simulink model "soc_dvbs2_hostUDPReceive"  (R2025b)
settings: Solver=VariableStepAuto  StartTime=0.0  StopTime=inf  RelTol=1e-3
values from neighbouring files (symbols this model uses):
  Rsym = 4e6    (= 4000000)    [soc_dvbs2_init.m]
libraries: dspnetwork x2, hdlsllib x2
settings Model: DataTypeOverride=Off  SimulationMode=accelerator  Creator=The MathWorks, Inc.  LastModifiedBy=The MathWorks, Inc.
settings SolverCC: MaxZcPerStep=1.0
settings OptimizationCC: BlockReduction=off  ConditionallyExecuteInputs=off  DefaultParameterBehavior=Inlined  ReuseModelBlockBuffer=off
settings DebuggingCC: AlgebraicLoopMsg=error  SingleTaskRateTransMsg=error  UnconnectedInputMsg=warning  UnconnectedOutputMsg=warning  UnconnectedLineMsg=warning  SubsystemReferenceDiagnosticForUnitTest=warning
settings HardwareCC: ProdBitPerPointer=32.0  ProdBitPerSizeT=32.0  ProdBitPerPtrDiffT=32.0  ProdLargestAtomicFloat=None  ProdIntDivRoundTo=Undefined  ProdEndianess=Unspecified  ProdWordSize=32.0  ProdHWDeviceType=ASIC/FPGA->ASIC/FPGA  TargetBitPerLong=64.0  TargetBitPerPointer=64.0  TargetBitPerSizeT=64.0  TargetBitPerPtrDiffT=64.0  TargetLongLongMode=on  TargetIntDivRoundTo=Zero  TargetEndianess=LittleEndian  TargetWordSize=64.0  TargetHWDeviceType=Custom Processor->MATLAB Host Computer  ProdEqTarget=off
settings ModelReferenceCC: EnableRefExpFcnMdlSchedulingChecks=on
settings RTWCC: GPUComputeCapability=3.5  DLArmComputeVersion=19.05

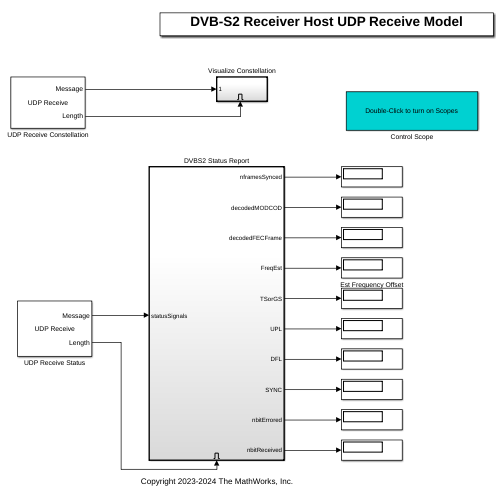
[thumbnail: Simulink's stored preview of the top-level diagram]
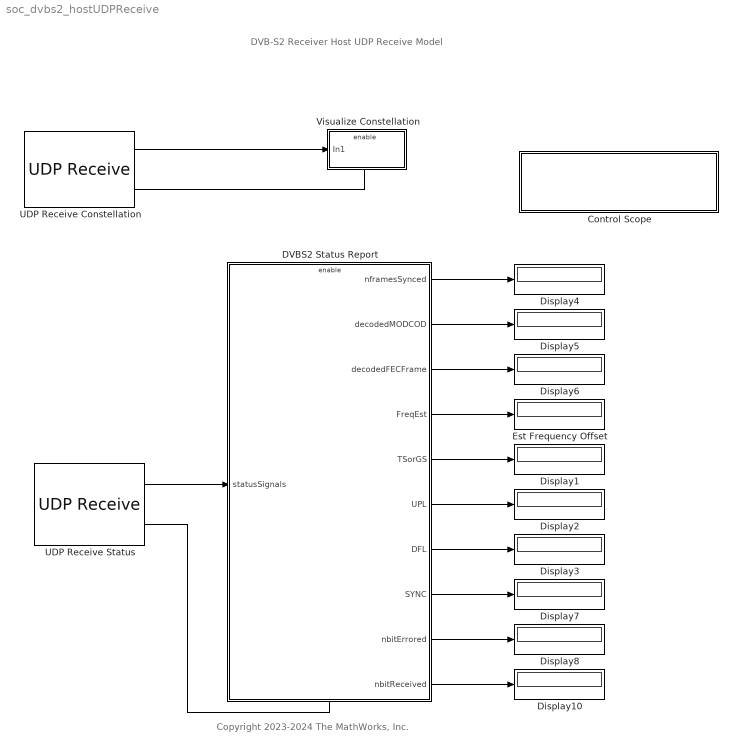
== system soc_dvbs2_hostUDPReceive ==
  note: DVB-S2 Receiver Host UDP Receive Model
  note: Copyright 2023-2024 The MathWorks, Inc.
  Control Scope : Subsystem
      settings: OpenFcn=|
      | ctrl = true;
      | hScopeConfig = get_param([gcs '/Visualize Constellation/Constellation Diagram'],'ScopeConfiguration');
      | hScopeConfig.Visible = ctrl;
      | clear hScopeConfig ctrl;
      mask Display: disp('Double-Click to turn on Scopes');
  DVBS2 Status Report : Subsystem
  Display{1..8,10} (9 alike) : Display
      Display7 settings: Format=hex (Stored Integer)
  Est Frequency Offset : Display
  UDP Receive Constellation : dspnetwork/UDP Receive  localURL='0.0.0.0'  localPort=25000  remoteURL='0.0.0.0'  remotePort=-1  recvBufferSize=8192  dims=2048  signalDatatype=uint32  isComplex=off  isVarSize=off  showBlockingTime=off  blockingTime=0  sampletime=1e-3  blockPlatform=[]
  UDP Receive Status : dspnetwork/UDP Receive  localURL='0.0.0.0'  localPort=25001  remoteURL='0.0.0.0'  remotePort=-1  recvBufferSize=8192  dims=10  signalDatatype=uint32  isComplex=off  isVarSize=off  showBlockingTime=off  blockingTime=0  sampletime=1e-3  blockPlatform=[]
  Visualize Constellation : Subsystem
  wires:
  DVBS2 Status Report/3(decodedFECFrame) -> Display6/1
  DVBS2 Status Report/4(FreqEst) -> Est Frequency Offset/1
  UDP Receive Constellation/1 -> Visualize Constellation/1(In1)
  UDP Receive Status/1 -> DVBS2 Status Report/1(statusSignals)
  DVBS2 Status Report/2(decodedMODCOD) -> Display5/1
  DVBS2 Status Report/1(nframesSynced) -> Display4/1
  UDP Receive Constellation/2 -> Visualize Constellation/Enable
  UDP Receive Status/2 -> DVBS2 Status Report/Enable
  DVBS2 Status Report/5(TSorGS) -> Display1/1
  DVBS2 Status Report/6(UPL) -> Display2/1
  DVBS2 Status Report/7(DFL) -> Display3/1
  DVBS2 Status Report/8(SYNC) -> Display7/1
  DVBS2 Status Report/9(nbitErrored) -> Display8/1
  DVBS2 Status Report/10(nbitReceived) -> Display10/1

== system soc_dvbs2_hostUDPReceive/Control Scope ==

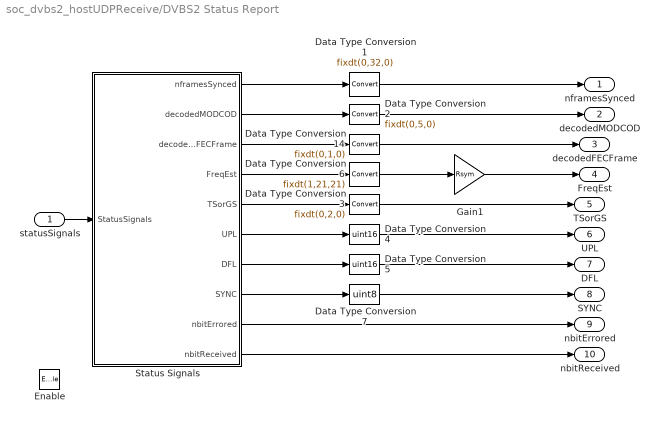
== system soc_dvbs2_hostUDPReceive/DVBS2 Status Report ==
  statusSignals : Inport
  Enable : EnablePort
  Data Type Conversion1 : DataTypeConversion  OutDataTypeStr=fixdt(0,32,0)  ConvertRealWorld=Stored Integer (SI)  SaturateOnIntegerOverflow=off  RndMeth=Floor
  Data Type Conversion14 : DataTypeConversion  OutDataTypeStr=fixdt(0,1,0)  ConvertRealWorld=Stored Integer (SI)  SaturateOnIntegerOverflow=off  RndMeth=Floor
  Data Type Conversion2 : DataTypeConversion  OutDataTypeStr=fixdt(0,5,0)  ConvertRealWorld=Stored Integer (SI)  SaturateOnIntegerOverflow=off  RndMeth=Floor
  Data Type Conversion3 : DataTypeConversion  OutDataTypeStr=fixdt(0,2,0)  ConvertRealWorld=Stored Integer (SI)  SaturateOnIntegerOverflow=off  RndMeth=Floor
  Data Type Conversion4 : DataTypeConversion  OutDataTypeStr=uint16  ConvertRealWorld=Stored Integer (SI)  SaturateOnIntegerOverflow=off  RndMeth=Floor
  Data Type Conversion5 : DataTypeConversion  OutDataTypeStr=uint16  ConvertRealWorld=Stored Integer (SI)  SaturateOnIntegerOverflow=off  RndMeth=Floor
  Data Type Conversion6 : DataTypeConversion  OutDataTypeStr=fixdt(1,21,21)  ConvertRealWorld=Stored Integer (SI)  SaturateOnIntegerOverflow=off  RndMeth=Floor
  Data Type Conversion7 : DataTypeConversion  OutDataTypeStr=uint8  ConvertRealWorld=Stored Integer (SI)  SaturateOnIntegerOverflow=off  RndMeth=Floor
  Gain1 : Gain  Gain=Rsym  ParamDataTypeStr=double
  Status Signals : Subsystem
  nframesSynced : Outport
  decodedMODCOD : Outport  Port=2
  decodedFECFrame : Outport  Port=3
  FreqEst : Outport  Port=4
  TSorGS : Outport  Port=5
  UPL : Outport  Port=6
  DFL : Outport  Port=7
  SYNC : Outport  Port=8
  nbitErrored : Outport  Port=9
  nbitReceived : Outport  Port=10
  wires:
  Data Type Conversion14/1 -> decodedFECFrame/1
  statusSignals/1 -> Status Signals/1(StatusSignals)
  Data Type Conversion2/1 -> decodedMODCOD/1
  Data Type Conversion6/1 -> Gain1/1
  Data Type Conversion1/1 -> nframesSynced/1
  Status Signals/2(decodedMODCOD) -> Data Type Conversion2/1
  Status Signals/1(nframesSynced) -> Data Type Conversion1/1
  Status Signals/3(decodedFECFrame) -> Data Type Conversion14/1
  Status Signals/4(FreqEst) -> Data Type Conversion6/1
  Gain1/1 -> FreqEst/1
  Status Signals/5(TSorGS) -> Data Type Conversion3/1
  Data Type Conversion3/1 -> TSorGS/1
  Status Signals/6(UPL) -> Data Type Conversion4/1
  Status Signals/7(DFL) -> Data Type Conversion5/1
  Data Type Conversion4/1 -> UPL/1
  Data Type Conversion5/1 -> DFL/1
  Status Signals/8(SYNC) -> Data Type Conversion7/1
  Data Type Conversion7/1 -> SYNC/1
  Status Signals/9(nbitErrored) -> nbitErrored/1
  Status Signals/10(nbitReceived) -> nbitReceived/1

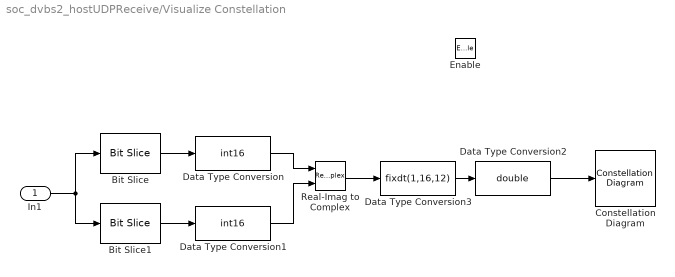
== system soc_dvbs2_hostUDPReceive/Visualize Constellation ==
  In1 : Inport
  Enable : EnablePort
  Bit Slice : hdlsllib/Logic and Bit Operations/Bit Slice  lidx=31  ridx=16
  Bit Slice1 : hdlsllib/Logic and Bit Operations/Bit Slice  lidx=15  ridx=0
  Constellation Diagram : ConstellationDiagram  WindowPosition=[390.000000,355.000000,402.000000,305.000000,]  ScopeFrameLocation=window  SymbolsToDisplaySource=Property  SymbolsToDisplay=1000  ReferenceConstellation="[0.70711+0.70711i        -0.70711+0.70711i        -0.70711-0.70711i         0.70711-0.70711i]"  XLimits=[-1.66,1.66]  YLimits=[-1.66,1.66]  AxesLimits=[-1.66,1.66]  DefaultConfigurationName=comm.scopes.ConstellationDiagramBlockCfg
  Data Type Conversion : DataTypeConversion  OutDataTypeStr=int16  ConvertRealWorld=Stored Integer (SI)  SaturateOnIntegerOverflow=off  RndMeth=Floor
  Data Type Conversion1 : DataTypeConversion  OutDataTypeStr=int16  ConvertRealWorld=Stored Integer (SI)  SaturateOnIntegerOverflow=off  RndMeth=Floor
  Data Type Conversion2 : DataTypeConversion  OutDataTypeStr=double  SaturateOnIntegerOverflow=off  RndMeth=Floor
  Data Type Conversion3 : DataTypeConversion  OutDataTypeStr=fixdt(1,16,12)  ConvertRealWorld=Stored Integer (SI)  SaturateOnIntegerOverflow=off  RndMeth=Floor
  Real-Imag to Complex : RealImagToComplex
  wires:
  Data Type Conversion3/1 -> Data Type Conversion2/1
  Bit Slice/1 -> Data Type Conversion/1
  In1/1 -> Bit Slice1/1, Bit Slice/1
  Bit Slice1/1 -> Data Type Conversion1/1
  Data Type Conversion/1 -> Real-Imag to Complex/1
  Data Type Conversion1/1 -> Real-Imag to Complex/2
  Real-Imag to Complex/1 -> Data Type Conversion3/1
  Data Type Conversion2/1 -> Constellation Diagram/1

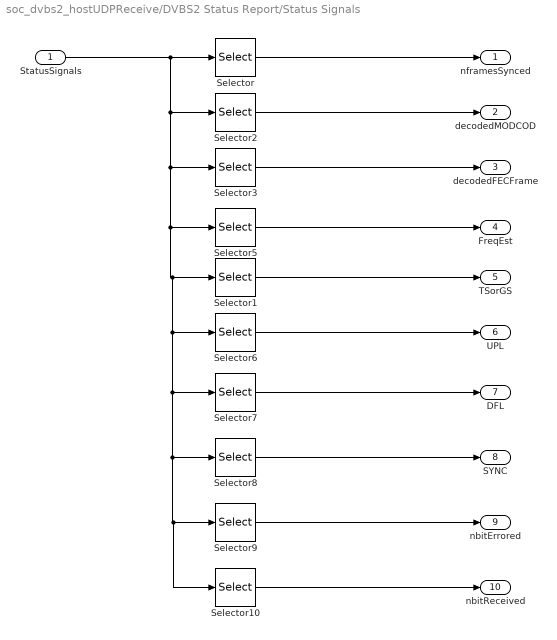
== system soc_dvbs2_hostUDPReceive/DVBS2 Status Report/Status Signals ==
  StatusSignals : Inport
  Selector : Selector  InputPortWidth=10  IndexOptions=Index vector (dialog)  Indices=[1]  OutputSizes=1
  Selector1 : Selector  InputPortWidth=10  IndexOptions=Index vector (dialog)  Indices=[5]  OutputSizes=1
  Selector10 : Selector  InputPortWidth=10  IndexOptions=Index vector (dialog)  Indices=[10]  OutputSizes=1
  Selector2 : Selector  InputPortWidth=10  IndexOptions=Index vector (dialog)  Indices=[2]  OutputSizes=1
  Selector3 : Selector  InputPortWidth=10  IndexOptions=Index vector (dialog)  Indices=[3]  OutputSizes=1
  Selector5 : Selector  InputPortWidth=10  IndexOptions=Index vector (dialog)  Indices=[4]  OutputSizes=1
  Selector6 : Selector  InputPortWidth=10  IndexOptions=Index vector (dialog)  Indices=[6]  OutputSizes=1
  Selector7 : Selector  InputPortWidth=10  IndexOptions=Index vector (dialog)  Indices=[7]  OutputSizes=1
  Selector8 : Selector  InputPortWidth=10  IndexOptions=Index vector (dialog)  Indices=[8]  OutputSizes=1
  Selector9 : Selector  InputPortWidth=10  IndexOptions=Index vector (dialog)  Indices=[9]  OutputSizes=1
  nframesSynced : Outport
  decodedMODCOD : Outport  Port=2
  decodedFECFrame : Outport  Port=3
  FreqEst : Outport  Port=4
  TSorGS : Outport  Port=5
  UPL : Outport  Port=6
  DFL : Outport  Port=7
  SYNC : Outport  Port=8
  nbitErrored : Outport  Port=9
  nbitReceived : Outport  Port=10
  wires:
  Selector3/1 -> decodedFECFrame/1
  Selector2/1 -> decodedMODCOD/1
  Selector5/1 -> FreqEst/1
  Selector/1 -> nframesSynced/1
  StatusSignals/1 -> Selector3/1, Selector8/1, Selector10/1, Selector9/1, Selector7/1, Selector6/1, Selector1/1, Selector5/1, Selector2/1, Selector/1
  Selector1/1 -> TSorGS/1
  Selector7/1 -> DFL/1
  Selector6/1 -> UPL/1
  Selector8/1 -> SYNC/1
  Selector9/1 -> nbitErrored/1
  Selector10/1 -> nbitReceived/1
